simulink model "I_for_8_coils_diagonal_motion"  (R2021b)
settings: Solver=FixedStepAuto  StartTime=4400e-6  StopTime=14760e-6  FixedStep=50e-6  RelTol=1e-3
libraries: simulink x12
(part 2 of 6)

== matlab function I_for_8_coils_diagonal_motion/Left_Coil/Right_Coil/Outer5 Coils/Coil-8 ==
  data: dxp_dz output; x_new input; y_new input; z_new input; dxn_dz output; dyp_dz output; dyn_dz output
function  [dxp_dz, dxn_dz, dyp_dz, dyn_dz] = current(x_new, y_new, z_new)

g = 415e-6;     %Coil spacing
m0 = 4*pi*1e-7;
radius = 3e-3;%m
height = 1e-3;%m
Magentization = 1.45; %T
vol_cy = pi*radius^2*height; % If Object is Cylinder, vol in m^3
% vol_sp = (4/3)*(pi * radius^3); % If Object is Sphere, vol in m^3

k = 0.4e-3; %additional length added to wires, to get concentric coil
%--------%--------%--------%--------%--------%--------%--------%----------
% Line along y - axis
%-%--------%--------%--------%--------%--------%--------%--------%--------
yp1_1 = -0.6e-3 - 7*k;
yp2_1 = 0.6e-3 + 7*k;
yn1_1 = -0.8e-3 - 7*k;
yn2_1 = 0.8e-3 + 7*k;
a_xp_1 = 8*g;  
a_xn_1 = -8*g;

k_yp_1 = 1/(4*pi*((a_xp_1-x_new)^2+z_new^2));
k_1yp_1 = (yp2_1-y_new)/((yp2_1-y_new)^2+(a_xp_1-x_new)^2+z_new^2)^0.5;
k_2yp_1 = (yp1_1-y_new)/((yp1_1-y_new)^2+(a_xp_1-x_new)^2+z_new^2)^0.5;

k_1yp_3 = (yp2_1-y_new)/((yp2_1-y_new)^2+(a_xp_1-x_new)^2+z_new^2)^1.5;
k_2yp_3 = (yp1_1-y_new)/((yp1_1-y_new)^2+(a_xp_1-x_new)^2+z_new^2)^1.5;

k_yn_1 = 1/(4*pi*((a_xn_1-x_new)^2+z_new^2));
k_1yn_1 = (yn2_1-y_new)/((yn2_1-y_new)^2+(a_xn_1-x_new)^2+z_new^2)^0.5;
k_2yn_1 = (yn1_1-y_new)/((yn1_1-y_new)^2+(a_xn_1-x_new)^2+z_new^2)^0.5;

k_1yn_3 = (yn2_1-y_new)/((yn2_1-y_new)^2+(a_xn_1-x_new)^2+z_new^2)^1.5;
k_2yn_3 = (yn1_1-y_new)/((yn1_1-y_new)^2+(a_xn_1-x_new)^2+z_new^2)^1.5;


hyp_z_1 = (k_yp_1) *m0;
hyp_z1_1 = (k_1yp_1 - k_2yp_1)*(-1);
hyp_z2_1 = (k_yp_1*(k_1yp_1 - k_2yp_1)*(z_new^2))*4*pi*2;
hyp_z3_1 = (k_1yp_3 - k_2yp_3)*(z_new^2);
dxp_dz = hyp_z_1*(hyp_z1_1 + hyp_z2_1 + hyp_z3_1);


hyn_z_1 = (k_yn_1)* m0*(-1);
hyn_z1_1 = (k_1yn_1 - k_2yn_1)*(-1);
hyn_z2_1 = (k_yn_1*(k_1yn_1 - k_2yn_1)*(z_new^2))*4*pi*2;
hyn_z3_1 = (k_1yn_3 - k_2yn_3)*(z_new^2);
dxn_dz = hyn_z_1*(hyn_z1_1 + hyn_z2_1 + hyn_z3_1);

%--------%--------%--------%--------%--------%--------%--------%----------
% Line along x - axis
%-%--------%--------%--------%--------%a--------%--------%--------%--------
xp1_1 = -0.8e-3 - 7*k;
xp2_1 = 0.8e-3 + 7*k;
xn1_1 = -1e-3 - 7*k;
xn2_1 = 1e-3 + 7*k;
a_yp_1 = 3.475;          %Distance of coil from (0,0)
a_yn_1 = -3.475;

k_xp_1 = 1/(4*pi*((a_yp_1-y_new)^2+z_new^2));
k_1xp_1 = (xp2_1-x_new)/((xp2_1-x_new)^2+(a_yp_1-y_new)^2+z_new^2)^0.5;
k_2xp_1 = (xp1_1-x_new)/((xp1_1-x_new)^2+(a_yp_1-y_new)^2+z_new^2)^0.5;

k_xn_1 = 1/(4*pi*((a_yn_1-y_new)^2+z_new^2));
k_1xn_1 = (xn2_1-x_new)/((xn2_1-x_new)^2+(a_yn_1-y_new)^2+z_new^2)^0.5;
k_2xn_1 = (xn1_1-x_new)/((xn1_1-x_new)^2+(a_yn_1-y_new)^2+z_new^2)^0.5;

k_1xp_3 = (xp2_1-x_new)/((xp2_1-x_new)^2+(a_yp_1-y_new)^2+z_new^2)^1.5;
k_2xp_3 = (xp1_1-x_new)/((xp1_1-x_new)^2+(a_yp_1-y_new)^2+z_new^2)^1.5;

k_1xn_3 = (xn2_1-x_new)/((xn2_1-x_new)^2+(a_yn_1-y_new)^2+z_new^2)^1.5;
k_2xn_3 = (xn1_1-x_new)/((xn1_1-x_new)^2+(a_yn_1-y_new)^2+z_new^2)^1.5;


hxp_z_1 = (k_xp_1)*m0;
hxp_z1_1 = (k_1xp_1 - k_2xp_1)*(-1);
hxp_z2_1 = (k_xp_1*(k_1xp_1 - k_2xp_1)*(z_new^2))*4*pi*2;
hxp_z3_1 = (k_1xp_3 - k_2xp_3)*(z_new^2);
dyp_dz = hxp_z_1*(hxp_z1_1 + hxp_z2_1 + hxp_z3_1);


hxn_z_1 = (k_xn_1)*m0*(-1);
hxn_z1_1 = (k_1xn_1 - k_2xn_1)*(-1);
hxn_z2_1 = (k_xn_1*(k_1xn_1 - k_2xn_1)*(z_new^2))*4*pi*2;
hxn_z3_1 = (k_1xn_3 - k_2xn_3)*(z_new^2);
dyn_dz = hxn_z_1*(hxn_z1_1 + hxn_z2_1 + hxn_z3_1);

end

== matlab function I_for_8_coils_diagonal_motion/Left_Bottom_Coil/Required Current in Coil1 ==
  data: F_xz_1 input; F_yz_1 input; I output; dxp_dz input; dxn_dz input; dyp_dz input; dyn_dz input; x_new input; y_new input
function  I = current(F_xz_1, F_yz_1,dxp_dz, dxn_dz, dyp_dz, dyn_dz, x_new, y_new)
radius = 3e-3;%m
height = 1e-3;%m
Magentization = 1.45; %T
m0 = 4*pi*10e-7;
vol_cy = pi*radius^2*height; % If Object is Cylinder, vol in m^3
if F_yz_1 == 0 && x_new ~= 0
        I = (F_xz_1/ (dxp_dz + dxn_dz))* m0/ (vol_cy * Magentization);
    elseif F_xz_1 == 0 && y_new ~= 0
        I = (F_yz_1 / (dyp_dz + dyn_dz))* m0/ (vol_cy * Magentization);
    elseif F_xz_1== 0 && F_yz_1 == 0 
        I = 0;
    else
        I = (F_xz_1/ (dxp_dz + dxn_dz)+  F_yz_1 / (dyp_dz + dyn_dz))* m0/ (vol_cy * Magentization);
end
end

== matlab function I_for_8_coils_diagonal_motion/Left_Coil/Right_Coil/Outer5 Coils/Coil-10 ==
  data: dxp_dz output; x_new input; y_new input; z_new input; dxn_dz output; dyp_dz output; dyn_dz output
function  [dxp_dz, dxn_dz, dyp_dz, dyn_dz] = current(x_new, y_new, z_new)

g = 412e-6;     %Coil spacing
m0 = 4*pi*1e-7;
radius = 3e-3;%m
height = 1e-3;%m
Magentization = 1.45; %T
vol_cy = pi*radius^2*height; % If Object is Cylinder, vol in m^3
% vol_sp = (4/3)*(pi * radius^3); % If Object is Sphere, vol in m^3

k = 0.4e-3; %additional length added to wires, to get concentric coil
%--------%--------%--------%--------%--------%--------%--------%----------
% Line along y - axis
%-%--------%--------%--------%--------%--------%--------%--------%--------
yp1_1 = -0.6e-3 - 9*k;
yp2_1 = 0.6e-3 + 9*k;
yn1_1 = -0.8e-3 - 9*k;
yn2_1 = 0.8e-3 + 9*k;
a_xp_1 = 10*g;  
a_xn_1 = -10*g;

k_yp_1 = 1/(4*pi*((a_xp_1-x_new)^2+z_new^2));
k_1yp_1 = (yp2_1-y_new)/((yp2_1-y_new)^2+(a_xp_1-x_new)^2+z_new^2)^0.5;
k_2yp_1 = (yp1_1-y_new)/((yp1_1-y_new)^2+(a_xp_1-x_new)^2+z_new^2)^0.5;

k_1yp_3 = (yp2_1-y_new)/((yp2_1-y_new)^2+(a_xp_1-x_new)^2+z_new^2)^1.5;
k_2yp_3 = (yp1_1-y_new)/((yp1_1-y_new)^2+(a_xp_1-x_new)^2+z_new^2)^1.5;

k_yn_1 = 1/(4*pi*((a_xn_1-x_new)^2+z_new^2));
k_1yn_1 = (yn2_1-y_new)/((yn2_1-y_new)^2+(a_xn_1-x_new)^2+z_new^2)^0.5;
k_2yn_1 = (yn1_1-y_new)/((yn1_1-y_new)^2+(a_xn_1-x_new)^2+z_new^2)^0.5;

k_1yn_3 = (yn2_1-y_new)/((yn2_1-y_new)^2+(a_xn_1-x_new)^2+z_new^2)^1.5;
k_2yn_3 = (yn1_1-y_new)/((yn1_1-y_new)^2+(a_xn_1-x_new)^2+z_new^2)^1.5;


hyp_z_1 = (k_yp_1) *m0;
hyp_z1_1 = (k_1yp_1 - k_2yp_1)*(-1);
hyp_z2_1 = (k_yp_1*(k_1yp_1 - k_2yp_1)*(z_new^2))*4*pi*2;
hyp_z3_1 = (k_1yp_3 - k_2yp_3)*(z_new^2);
dxp_dz = hyp_z_1*(hyp_z1_1 + hyp_z2_1 + hyp_z3_1);


hyn_z_1 = (k_yn_1)* m0*(-1);
hyn_z1_1 = (k_1yn_1 - k_2yn_1)*(-1);
hyn_z2_1 = (k_yn_1*(k_1yn_1 - k_2yn_1)*(z_new^2))*4*pi*2;
hyn_z3_1 = (k_1yn_3 - k_2yn_3)*(z_new^2);
dxn_dz = hyn_z_1*(hyn_z1_1 + hyn_z2_1 + hyn_z3_1);

%--------%--------%--------%--------%--------%--------%--------%----------
% Line along x - axis
%-%--------%--------%--------%--------%a--------%--------%--------%--------
xp1_1 = -0.8e-3 - 9*k;
xp2_1 = 0.8e-3 + 9*k;
xn1_1 = -1e-3 - 9*k;
xn2_1 = 1e-3 + 9*k;
a_yp_1 = 4.275;          %Distance of coil from (0,0)
a_yn_1 = -4.275;

k_xp_1 = 1/(4*pi*((a_yp_1-y_new)^2+z_new^2));
k_1xp_1 = (xp2_1-x_new)/((xp2_1-x_new)^2+(a_yp_1-y_new)^2+z_new^2)^0.5;
k_2xp_1 = (xp1_1-x_new)/((xp1_1-x_new)^2+(a_yp_1-y_new)^2+z_new^2)^0.5;

k_xn_1 = 1/(4*pi*((a_yn_1-y_new)^2+z_new^2));
k_1xn_1 = (xn2_1-x_new)/((xn2_1-x_new)^2+(a_yn_1-y_new)^2+z_new^2)^0.5;
k_2xn_1 = (xn1_1-x_new)/((xn1_1-x_new)^2+(a_yn_1-y_new)^2+z_new^2)^0.5;

k_1xp_3 = (xp2_1-x_new)/((xp2_1-x_new)^2+(a_yp_1-y_new)^2+z_new^2)^1.5;
k_2xp_3 = (xp1_1-x_new)/((xp1_1-x_new)^2+(a_yp_1-y_new)^2+z_new^2)^1.5;

k_1xn_3 = (xn2_1-x_new)/((xn2_1-x_new)^2+(a_yn_1-y_new)^2+z_new^2)^1.5;
k_2xn_3 = (xn1_1-x_new)/((xn1_1-x_new)^2+(a_yn_1-y_new)^2+z_new^2)^1.5;


hxp_z_1 = (k_xp_1)*m0;
hxp_z1_1 = (k_1xp_1 - k_2xp_1)*(-1);
hxp_z2_1 = (k_xp_1*(k_1xp_1 - k_2xp_1)*(z_new^2))*4*pi*2;
hxp_z3_1 = (k_1xp_3 - k_2xp_3)*(z_new^2);
dyp_dz = hxp_z_1*(hxp_z1_1 + hxp_z2_1 + hxp_z3_1);


hxn_z_1 = (k_xn_1)*m0*(-1);
hxn_z1_1 = (k_1xn_1 - k_2xn_1)*(-1);
hxn_z2_1 = (k_xn_1*(k_1xn_1 - k_2xn_1)*(z_new^2))*4*pi*2;
hxn_z3_1 = (k_1xn_3 - k_2xn_3)*(z_new^2);
dyn_dz = hxn_z_1*(hxn_z1_1 + hxn_z2_1 + hxn_z3_1);

end

== matlab function I_for_8_coils_diagonal_motion/Left_Bottom_Coil/Left_Coil/Inner 5 Coils/Coil-1 ==
  data: dxp_dz output; x_new input; y_new input; z_new input; dxn_dz output; dyp_dz output; dyn_dz output
function  [dxp_dz, dxn_dz, dyp_dz, dyn_dz] = current(x_new, y_new, z_new)

g = 520e-6;     %Coil spacing
m0 = 4*pi*1e-7;
radius = 3e-3;%m
height = 1e-3;%m
Magentization = 1.45; %T
vol_cy = pi*radius^2*height; % If Object is Cylinder, vol in m^3
% vol_sp = (4/3)*(pi * radius^3); % If Object is Sphere, vol in m^3

k = 0.4e-3; %additional length added to wires, to get concentric coil
%--------%--------%--------%--------%--------%--------%--------%----------
% Line along y - axis
%-%--------%--------%--------%--------%--------%--------%--------%--------
yp1_1 = -0.6e-3 ;
yp2_1 = 0.6e-3 ;
yn1_1 = -0.8e-3 ;
yn2_1 = 0.8e-3;
a_xp_1 = g;  
a_xn_1 = -g;

k_yp_1 = 1/(4*pi*((a_xp_1-x_new)^2+z_new^2));
k_1yp_1 = (yp2_1-y_new)/((yp2_1-y_new)^2+(a_xp_1-x_new)^2+z_new^2)^0.5;
k_2yp_1 = (yp1_1-y_new)/((yp1_1-y_new)^2+(a_xp_1-x_new)^2+z_new^2)^0.5;

k_1yp_3 = (yp2_1-y_new)/((yp2_1-y_new)^2+(a_xp_1-x_new)^2+z_new^2)^1.5;
k_2yp_3 = (yp1_1-y_new)/((yp1_1-y_new)^2+(a_xp_1-x_new)^2+z_new^2)^1.5;

k_yn_1 = 1/(4*pi*((a_xn_1-x_new)^2+z_new^2));
k_1yn_1 = (yn2_1-y_new)/((yn2_1-y_new)^2+(a_xn_1-x_new)^2+z_new^2)^0.5;
k_2yn_1 = (yn1_1-y_new)/((yn1_1-y_new)^2+(a_xn_1-x_new)^2+z_new^2)^0.5;

k_1yn_3 = (yn2_1-y_new)/((yn2_1-y_new)^2+(a_xn_1-x_new)^2+z_new^2)^1.5;
k_2yn_3 = (yn1_1-y_new)/((yn1_1-y_new)^2+(a_xn_1-x_new)^2+z_new^2)^1.5;


hyp_z_1 = (k_yp_1) *m0;
hyp_z1_1 = (k_1yp_1 - k_2yp_1)*(-1);
hyp_z2_1 = (k_yp_1*(k_1yp_1 - k_2yp_1)*(z_new^2))*4*pi*2;
hyp_z3_1 = (k_1yp_3 - k_2yp_3)*(z_new^2);
dxp_dz = hyp_z_1*(hyp_z1_1 + hyp_z2_1 + hyp_z3_1);


hyn_z_1 = (k_yn_1)* m0*(-1);
hyn_z1_1 = (k_1yn_1 - k_2yn_1)*(-1);
hyn_z2_1 = (k_yn_1*(k_1yn_1 - k_2yn_1)*(z_new^2))*4*pi*2;
hyn_z3_1 = (k_1yn_3 - k_2yn_3)*(z_new^2);
dxn_dz = hyn_z_1*(hyn_z1_1 + hyn_z2_1 + hyn_z3_1);

%--------%--------%--------%--------%--------%--------%--------%----------
% Line along x - axis
%-%--------%--------%--------%--------%a--------%--------%--------%--------
xp1_1 = -0.8e-3 ;
xp2_1 = 0.8e-3 ;
xn1_1 = -1e-3 ;
xn2_1 = 1e-3 ;
a_yp_1 = 0.675;          %Distance of coil from (0,0)
a_yn_1 = -0.675;

k_xp_1 = 1/(4*pi*((a_yp_1-y_new)^2+z_new^2));
k_1xp_1 = (xp2_1-x_new)/((xp2_1-x_new)^2+(a_yp_1-y_new)^2+z_new^2)^0.5;
k_2xp_1 = (xp1_1-x_new)/((xp1_1-x_new)^2+(a_yp_1-y_new)^2+z_new^2)^0.5;

k_xn_1 = 1/(4*pi*((a_yn_1-y_new)^2+z_new^2));
k_1xn_1 = (xn2_1-x_new)/((xn2_1-x_new)^2+(a_yn_1-y_new)^2+z_new^2)^0.5;
k_2xn_1 = (xn1_1-x_new)/((xn1_1-x_new)^2+(a_yn_1-y_new)^2+z_new^2)^0.5;

k_1xp_3 = (xp2_1-x_new)/((xp2_1-x_new)^2+(a_yp_1-y_new)^2+z_new^2)^1.5;
k_2xp_3 = (xp1_1-x_new)/((xp1_1-x_new)^2+(a_yp_1-y_new)^2+z_new^2)^1.5;

k_1xn_3 = (xn2_1-x_new)/((xn2_1-x_new)^2+(a_yn_1-y_new)^2+z_new^2)^1.5;
k_2xn_3 = (xn1_1-x_new)/((xn1_1-x_new)^2+(a_yn_1-y_new)^2+z_new^2)^1.5;


hxp_z_1 = (k_xp_1)*m0;
hxp_z1_1 = (k_1xp_1 - k_2xp_1)*(-1);
hxp_z2_1 = (k_xp_1*(k_1xp_1 - k_2xp_1)*(z_new^2))*4*pi*2;
hxp_z3_1 = (k_1xp_3 - k_2xp_3)*(z_new^2);
dyp_dz = hxp_z_1*(hxp_z1_1 + hxp_z2_1 + hxp_z3_1);


hxn_z_1 = (k_xn_1)*m0*(-1);
hxn_z1_1 = (k_1xn_1 - k_2xn_1)*(-1);
hxn_z2_1 = (k_xn_1*(k_1xn_1 - k_2xn_1)*(z_new^2))*4*pi*2;
hxn_z3_1 = (k_1xn_3 - k_2xn_3)*(z_new^2);
dyn_dz = hxn_z_1*(hxn_z1_1 + hxn_z2_1 + hxn_z3_1);

end

== matlab function I_for_8_coils_diagonal_motion/Left_Bottom_Coil/Left_Coil/Inner 5 Coils/Coil-2 ==
  data: dxp_dz output; x_new input; y_new input; z_new input; dxn_dz output; dyp_dz output; dyn_dz output
function  [dxp_dz, dxn_dz, dyp_dz, dyn_dz] = current(x_new, y_new, z_new)

g = 460e-6;     %Coil spacing
m0 = 4*pi*1e-7;
radius = 3e-3;%m
height = 1e-3;%m
Magentization = 1.45; %T
vol_cy = pi*radius^2*height; % If Object is Cylinder, vol in m^3
% vol_sp = (4/3)*(pi * radius^3); % If Object is Sphere, vol in m^3

k = 0.4e-3; %additional length added to wires, to get concentric coil
%--------%--------%--------%--------%--------%--------%--------%----------
% Line along y - axis
%-%--------%--------%--------%--------%--------%--------%--------%--------
yp1_1 = -0.6e-3 - k;
yp2_1 = 0.6e-3 + k;
yn1_1 = -0.8e-3 - k;
yn2_1 = 0.8e-3 + k;
a_xp_1 = 2*g;  
a_xn_1 = -2*g;

k_yp_1 = 1/(4*pi*((a_xp_1-x_new)^2+z_new^2));
k_1yp_1 = (yp2_1-y_new)/((yp2_1-y_new)^2+(a_xp_1-x_new)^2+z_new^2)^0.5;
k_2yp_1 = (yp1_1-y_new)/((yp1_1-y_new)^2+(a_xp_1-x_new)^2+z_new^2)^0.5;

k_1yp_3 = (yp2_1-y_new)/((yp2_1-y_new)^2+(a_xp_1-x_new)^2+z_new^2)^1.5;
k_2yp_3 = (yp1_1-y_new)/((yp1_1-y_new)^2+(a_xp_1-x_new)^2+z_new^2)^1.5;

k_yn_1 = 1/(4*pi*((a_xn_1-x_new)^2+z_new^2));
k_1yn_1 = (yn2_1-y_new)/((yn2_1-y_new)^2+(a_xn_1-x_new)^2+z_new^2)^0.5;
k_2yn_1 = (yn1_1-y_new)/((yn1_1-y_new)^2+(a_xn_1-x_new)^2+z_new^2)^0.5;

k_1yn_3 = (yn2_1-y_new)/((yn2_1-y_new)^2+(a_xn_1-x_new)^2+z_new^2)^1.5;
k_2yn_3 = (yn1_1-y_new)/((yn1_1-y_new)^2+(a_xn_1-x_new)^2+z_new^2)^1.5;


hyp_z_1 = (k_yp_1) *m0;
hyp_z1_1 = (k_1yp_1 - k_2yp_1)*(-1);
hyp_z2_1 = (k_yp_1*(k_1yp_1 - k_2yp_1)*(z_new^2))*4*pi*2;
hyp_z3_1 = (k_1yp_3 - k_2yp_3)*(z_new^2);
dxp_dz = hyp_z_1*(hyp_z1_1 + hyp_z2_1 + hyp_z3_1);


hyn_z_1 = (k_yn_1)* m0*(-1);
hyn_z1_1 = (k_1yn_1 - k_2yn_1)*(-1);
hyn_z2_1 = (k_yn_1*(k_1yn_1 - k_2yn_1)*(z_new^2))*4*pi*2;
hyn_z3_1 = (k_1yn_3 - k_2yn_3)*(z_new^2);
dxn_dz = hyn_z_1*(hyn_z1_1 + hyn_z2_1 + hyn_z3_1);

%--------%--------%--------%--------%--------%--------%--------%----------
% Line along x - axis
%-%--------%--------%--------%--------%a--------%--------%--------%--------
xp1_1 = -0.8e-3 - k;
xp2_1 = 0.8e-3 + k;
xn1_1 = -1e-3 - k;
xn2_1 = 1e-3 + k;
a_yp_1 = 1.075;          %Distance of coil from (0,0)
a_yn_1 = -1.075;

k_xp_1 = 1/(4*pi*((a_yp_1-y_new)^2+z_new^2));
k_1xp_1 = (xp2_1-x_new)/((xp2_1-x_new)^2+(a_yp_1-y_new)^2+z_new^2)^0.5;
k_2xp_1 = (xp1_1-x_new)/((xp1_1-x_new)^2+(a_yp_1-y_new)^2+z_new^2)^0.5;

k_xn_1 = 1/(4*pi*((a_yn_1-y_new)^2+z_new^2));
k_1xn_1 = (xn2_1-x_new)/((xn2_1-x_new)^2+(a_yn_1-y_new)^2+z_new^2)^0.5;
k_2xn_1 = (xn1_1-x_new)/((xn1_1-x_new)^2+(a_yn_1-y_new)^2+z_new^2)^0.5;

k_1xp_3 = (xp2_1-x_new)/((xp2_1-x_new)^2+(a_yp_1-y_new)^2+z_new^2)^1.5;
k_2xp_3 = (xp1_1-x_new)/((xp1_1-x_new)^2+(a_yp_1-y_new)^2+z_new^2)^1.5;

k_1xn_3 = (xn2_1-x_new)/((xn2_1-x_new)^2+(a_yn_1-y_new)^2+z_new^2)^1.5;
k_2xn_3 = (xn1_1-x_new)/((xn1_1-x_new)^2+(a_yn_1-y_new)^2+z_new^2)^1.5;


hxp_z_1 = (k_xp_1)*m0;
hxp_z1_1 = (k_1xp_1 - k_2xp_1)*(-1);
hxp_z2_1 = (k_xp_1*(k_1xp_1 - k_2xp_1)*(z_new^2))*4*pi*2;
hxp_z3_1 = (k_1xp_3 - k_2xp_3)*(z_new^2);
dyp_dz = hxp_z_1*(hxp_z1_1 + hxp_z2_1 + hxp_z3_1);


hxn_z_1 = (k_xn_1)*m0*(-1);
hxn_z1_1 = (k_1xn_1 - k_2xn_1)*(-1);
hxn_z2_1 = (k_xn_1*(k_1xn_1 - k_2xn_1)*(z_new^2))*4*pi*2;
hxn_z3_1 = (k_1xn_3 - k_2xn_3)*(z_new^2);
dyn_dz = hxn_z_1*(hxn_z1_1 + hxn_z2_1 + hxn_z3_1);

end

== matlab function I_for_8_coils_diagonal_motion/Left_Bottom_Coil/Left_Coil/Inner 5 Coils/Coil-3 ==
  data: dxp_dz output; x_new input; y_new input; z_new input; dxn_dz output; dyp_dz output; dyn_dz output
function  [dxp_dz, dxn_dz, dyp_dz, dyn_dz] = current(x_new, y_new, z_new)

g = 440e-6;     %Coil spacing
m0 = 4*pi*1e-7;
radius = 3e-3;%m
height = 1e-3;%m
Magentization = 1.45; %T
vol_cy = pi*radius^2*height; % If Object is Cylinder, vol in m^3
% vol_sp = (4/3)*(pi * radius^3); % If Object is Sphere, vol in m^3

k = 0.4e-3; %additional length added to wires, to get concentric coil
%--------%--------%--------%--------%--------%--------%--------%----------
% Line along y - axis
%-%--------%--------%--------%--------%--------%--------%--------%--------
yp1_1 = -0.6e-3 - 2*k;
yp2_1 = 0.6e-3 + 2*k;
yn1_1 = -0.8e-3 - 2*k;
yn2_1 = 0.8e-3 + 2*k;
a_xp_1 = 3*g;  
a_xn_1 = -3*g;

k_yp_1 = 1/(4*pi*((a_xp_1-x_new)^2+z_new^2));
k_1yp_1 = (yp2_1-y_new)/((yp2_1-y_new)^2+(a_xp_1-x_new)^2+z_new^2)^0.5;
k_2yp_1 = (yp1_1-y_new)/((yp1_1-y_new)^2+(a_xp_1-x_new)^2+z_new^2)^0.5;

k_1yp_3 = (yp2_1-y_new)/((yp2_1-y_new)^2+(a_xp_1-x_new)^2+z_new^2)^1.5;
k_2yp_3 = (yp1_1-y_new)/((yp1_1-y_new)^2+(a_xp_1-x_new)^2+z_new^2)^1.5;

k_yn_1 = 1/(4*pi*((a_xn_1-x_new)^2+z_new^2));
k_1yn_1 = (yn2_1-y_new)/((yn2_1-y_new)^2+(a_xn_1-x_new)^2+z_new^2)^0.5;
k_2yn_1 = (yn1_1-y_new)/((yn1_1-y_new)^2+(a_xn_1-x_new)^2+z_new^2)^0.5;

k_1yn_3 = (yn2_1-y_new)/((yn2_1-y_new)^2+(a_xn_1-x_new)^2+z_new^2)^1.5;
k_2yn_3 = (yn1_1-y_new)/((yn1_1-y_new)^2+(a_xn_1-x_new)^2+z_new^2)^1.5;


hyp_z_1 = (k_yp_1) *m0;
hyp_z1_1 = (k_1yp_1 - k_2yp_1)*(-1);
hyp_z2_1 = (k_yp_1*(k_1yp_1 - k_2yp_1)*(z_new^2))*4*pi*2;
hyp_z3_1 = (k_1yp_3 - k_2yp_3)*(z_new^2);
dxp_dz = hyp_z_1*(hyp_z1_1 + hyp_z2_1 + hyp_z3_1);


hyn_z_1 = (k_yn_1)* m0*(-1);
hyn_z1_1 = (k_1yn_1 - k_2yn_1)*(-1);
hyn_z2_1 = (k_yn_1*(k_1yn_1 - k_2yn_1)*(z_new^2))*4*pi*2;
hyn_z3_1 = (k_1yn_3 - k_2yn_3)*(z_new^2);
dxn_dz = hyn_z_1*(hyn_z1_1 + hyn_z2_1 + hyn_z3_1);

%--------%--------%--------%--------%--------%--------%--------%----------
% Line along x - axis
%-%--------%--------%--------%--------%a--------%--------%--------%--------
xp1_1 = -0.8e-3 - 2*k;
xp2_1 = 0.8e-3 + 2*k;
xn1_1 = -1e-3 - 2*k;
xn2_1 = 1e-3 + 2*k;
a_yp_1 = 1.475;          %Distance of coil from (0,0)
a_yn_1 = -1.475;

k_xp_1 = 1/(4*pi*((a_yp_1-y_new)^2+z_new^2));
k_1xp_1 = (xp2_1-x_new)/((xp2_1-x_new)^2+(a_yp_1-y_new)^2+z_new^2)^0.5;
k_2xp_1 = (xp1_1-x_new)/((xp1_1-x_new)^2+(a_yp_1-y_new)^2+z_new^2)^0.5;

k_xn_1 = 1/(4*pi*((a_yn_1-y_new)^2+z_new^2));
k_1xn_1 = (xn2_1-x_new)/((xn2_1-x_new)^2+(a_yn_1-y_new)^2+z_new^2)^0.5;
k_2xn_1 = (xn1_1-x_new)/((xn1_1-x_new)^2+(a_yn_1-y_new)^2+z_new^2)^0.5;

k_1xp_3 = (xp2_1-x_new)/((xp2_1-x_new)^2+(a_yp_1-y_new)^2+z_new^2)^1.5;
k_2xp_3 = (xp1_1-x_new)/((xp1_1-x_new)^2+(a_yp_1-y_new)^2+z_new^2)^1.5;

k_1xn_3 = (xn2_1-x_new)/((xn2_1-x_new)^2+(a_yn_1-y_new)^2+z_new^2)^1.5;
k_2xn_3 = (xn1_1-x_new)/((xn1_1-x_new)^2+(a_yn_1-y_new)^2+z_new^2)^1.5;


hxp_z_1 = (k_xp_1)*m0;
hxp_z1_1 = (k_1xp_1 - k_2xp_1)*(-1);
hxp_z2_1 = (k_xp_1*(k_1xp_1 - k_2xp_1)*(z_new^2))*4*pi*2;
hxp_z3_1 = (k_1xp_3 - k_2xp_3)*(z_new^2);
dyp_dz = hxp_z_1*(hxp_z1_1 + hxp_z2_1 + hxp_z3_1);


hxn_z_1 = (k_xn_1)*m0*(-1);
hxn_z1_1 = (k_1xn_1 - k_2xn_1)*(-1);
hxn_z2_1 = (k_xn_1*(k_1xn_1 - k_2xn_1)*(z_new^2))*4*pi*2;
hxn_z3_1 = (k_1xn_3 - k_2xn_3)*(z_new^2);
dyn_dz = hxn_z_1*(hxn_z1_1 + hxn_z2_1 + hxn_z3_1);

end

== matlab function I_for_8_coils_diagonal_motion/Left_Bottom_Coil/Left_Coil/Inner 5 Coils/Coil-4 ==
  data: dxp_dz output; x_new input; y_new input; z_new input; dxn_dz output; dyp_dz output; dyn_dz output
function  [dxp_dz, dxn_dz, dyp_dz, dyn_dz] = current(x_new, y_new, z_new)

g = 430e-6;     %Coil spacing
m0 = 4*pi*1e-7;
radius = 3e-3;%m
height = 1e-3;%m
Magentization = 1.45; %T
vol_cy = pi*radius^2*height; % If Object is Cylinder, vol in m^3
% vol_sp = (4/3)*(pi * radius^3); % If Object is Sphere, vol in m^3

k = 0.4e-3; %additional length added to wires, to get concentric coil
%--------%--------%--------%--------%--------%--------%--------%----------
% Line along y - axis
%-%--------%--------%--------%--------%--------%--------%--------%--------
yp1_1 = -0.6e-3 - 3*k;
yp2_1 = 0.6e-3 + 3*k;
yn1_1 = -0.8e-3 - 3*k;
yn2_1 = 0.8e-3 + 3*k;
a_xp_1 = 4*g;  
a_xn_1 = -4*g;

k_yp_1 = 1/(4*pi*((a_xp_1-x_new)^2+z_new^2));
k_1yp_1 = (yp2_1-y_new)/((yp2_1-y_new)^2+(a_xp_1-x_new)^2+z_new^2)^0.5;
k_2yp_1 = (yp1_1-y_new)/((yp1_1-y_new)^2+(a_xp_1-x_new)^2+z_new^2)^0.5;

k_1yp_3 = (yp2_1-y_new)/((yp2_1-y_new)^2+(a_xp_1-x_new)^2+z_new^2)^1.5;
k_2yp_3 = (yp1_1-y_new)/((yp1_1-y_new)^2+(a_xp_1-x_new)^2+z_new^2)^1.5;

k_yn_1 = 1/(4*pi*((a_xn_1-x_new)^2+z_new^2));
k_1yn_1 = (yn2_1-y_new)/((yn2_1-y_new)^2+(a_xn_1-x_new)^2+z_new^2)^0.5;
k_2yn_1 = (yn1_1-y_new)/((yn1_1-y_new)^2+(a_xn_1-x_new)^2+z_new^2)^0.5;

k_1yn_3 = (yn2_1-y_new)/((yn2_1-y_new)^2+(a_xn_1-x_new)^2+z_new^2)^1.5;
k_2yn_3 = (yn1_1-y_new)/((yn1_1-y_new)^2+(a_xn_1-x_new)^2+z_new^2)^1.5;


hyp_z_1 = (k_yp_1) *m0;
hyp_z1_1 = (k_1yp_1 - k_2yp_1)*(-1);
hyp_z2_1 = (k_yp_1*(k_1yp_1 - k_2yp_1)*(z_new^2))*4*pi*2;
hyp_z3_1 = (k_1yp_3 - k_2yp_3)*(z_new^2);
dxp_dz = hyp_z_1*(hyp_z1_1 + hyp_z2_1 + hyp_z3_1);


hyn_z_1 = (k_yn_1)* m0*(-1);
hyn_z1_1 = (k_1yn_1 - k_2yn_1)*(-1);
hyn_z2_1 = (k_yn_1*(k_1yn_1 - k_2yn_1)*(z_new^2))*4*pi*2;
hyn_z3_1 = (k_1yn_3 - k_2yn_3)*(z_new^2);
dxn_dz = hyn_z_1*(hyn_z1_1 + hyn_z2_1 + hyn_z3_1);

%--------%--------%--------%--------%--------%--------%--------%----------
% Line along x - axis
%-%--------%--------%--------%--------%a--------%--------%--------%--------
xp1_1 = -0.8e-3 - 3*k;
xp2_1 = 0.8e-3 + 3*k;
xn1_1 = -1e-3 - 3*k;
xn2_1 = 1e-3 + 3*k;
a_yp_1 = 1.875;          %Distance of coil from (0,0)
a_yn_1 = -1.875;

k_xp_1 = 1/(4*pi*((a_yp_1-y_new)^2+z_new^2));
k_1xp_1 = (xp2_1-x_new)/((xp2_1-x_new)^2+(a_yp_1-y_new)^2+z_new^2)^0.5;
k_2xp_1 = (xp1_1-x_new)/((xp1_1-x_new)^2+(a_yp_1-y_new)^2+z_new^2)^0.5;

k_xn_1 = 1/(4*pi*((a_yn_1-y_new)^2+z_new^2));
k_1xn_1 = (xn2_1-x_new)/((xn2_1-x_new)^2+(a_yn_1-y_new)^2+z_new^2)^0.5;
k_2xn_1 = (xn1_1-x_new)/((xn1_1-x_new)^2+(a_yn_1-y_new)^2+z_new^2)^0.5;

k_1xp_3 = (xp2_1-x_new)/((xp2_1-x_new)^2+(a_yp_1-y_new)^2+z_new^2)^1.5;
k_2xp_3 = (xp1_1-x_new)/((xp1_1-x_new)^2+(a_yp_1-y_new)^2+z_new^2)^1.5;

k_1xn_3 = (xn2_1-x_new)/((xn2_1-x_new)^2+(a_yn_1-y_new)^2+z_new^2)^1.5;
k_2xn_3 = (xn1_1-x_new)/((xn1_1-x_new)^2+(a_yn_1-y_new)^2+z_new^2)^1.5;


hxp_z_1 = (k_xp_1)*m0;
hxp_z1_1 = (k_1xp_1 - k_2xp_1)*(-1);
hxp_z2_1 = (k_xp_1*(k_1xp_1 - k_2xp_1)*(z_new^2))*4*pi*2;
hxp_z3_1 = (k_1xp_3 - k_2xp_3)*(z_new^2);
dyp_dz = hxp_z_1*(hxp_z1_1 + hxp_z2_1 + hxp_z3_1);


hxn_z_1 = (k_xn_1)*m0*(-1);
hxn_z1_1 = (k_1xn_1 - k_2xn_1)*(-1);
hxn_z2_1 = (k_xn_1*(k_1xn_1 - k_2xn_1)*(z_new^2))*4*pi*2;
hxn_z3_1 = (k_1xn_3 - k_2xn_3)*(z_new^2);
dyn_dz = hxn_z_1*(hxn_z1_1 + hxn_z2_1 + hxn_z3_1);

end

== matlab function I_for_8_coils_diagonal_motion/Left_Bottom_Coil/Left_Coil/Inner 5 Coils/Coil-5 ==
  data: dxp_dz output; x_new input; y_new input; z_new input; dxn_dz output; dyp_dz output; dyn_dz output
function  [dxp_dz, dxn_dz, dyp_dz, dyn_dz] = current(x_new, y_new, z_new)

g = 424e-6;     %Coil spacing
m0 = 4*pi*1e-7;
radius = 3e-3;%m
height = 1e-3;%m
Magentization = 1.45; %T
vol_cy = pi*radius^2*height; % If Object is Cylinder, vol in m^3
% vol_sp = (4/3)*(pi * radius^3); % If Object is Sphere, vol in m^3

k = 0.4e-3; %additional length added to wires, to get concentric coil
%--------%--------%--------%--------%--------%--------%--------%----------
% Line along y - axis
%-%--------%--------%--------%--------%--------%--------%--------%--------
yp1_1 = -0.6e-3 - 4*k;
yp2_1 = 0.6e-3 + 4*k;
yn1_1 = -0.8e-3 - 4*k;
yn2_1 = 0.8e-3 + 4*k;
a_xp_1 = 5*g;  
a_xn_1 = -5*g;

k_yp_1 = 1/(4*pi*((a_xp_1-x_new)^2+z_new^2));
k_1yp_1 = (yp2_1-y_new)/((yp2_1-y_new)^2+(a_xp_1-x_new)^2+z_new^2)^0.5;
k_2yp_1 = (yp1_1-y_new)/((yp1_1-y_new)^2+(a_xp_1-x_new)^2+z_new^2)^0.5;

k_1yp_3 = (yp2_1-y_new)/((yp2_1-y_new)^2+(a_xp_1-x_new)^2+z_new^2)^1.5;
k_2yp_3 = (yp1_1-y_new)/((yp1_1-y_new)^2+(a_xp_1-x_new)^2+z_new^2)^1.5;

k_yn_1 = 1/(4*pi*((a_xn_1-x_new)^2+z_new^2));
k_1yn_1 = (yn2_1-y_new)/((yn2_1-y_new)^2+(a_xn_1-x_new)^2+z_new^2)^0.5;
k_2yn_1 = (yn1_1-y_new)/((yn1_1-y_new)^2+(a_xn_1-x_new)^2+z_new^2)^0.5;

k_1yn_3 = (yn2_1-y_new)/((yn2_1-y_new)^2+(a_xn_1-x_new)^2+z_new^2)^1.5;
k_2yn_3 = (yn1_1-y_new)/((yn1_1-y_new)^2+(a_xn_1-x_new)^2+z_new^2)^1.5;


hyp_z_1 = (k_yp_1) *m0;
hyp_z1_1 = (k_1yp_1 - k_2yp_1)*(-1);
hyp_z2_1 = (k_yp_1*(k_1yp_1 - k_2yp_1)*(z_new^2))*4*pi*2;
hyp_z3_1 = (k_1yp_3 - k_2yp_3)*(z_new^2);
dxp_dz = hyp_z_1*(hyp_z1_1 + hyp_z2_1 + hyp_z3_1);


hyn_z_1 = (k_yn_1)* m0*(-1);
hyn_z1_1 = (k_1yn_1 - k_2yn_1)*(-1);
hyn_z2_1 = (k_yn_1*(k_1yn_1 - k_2yn_1)*(z_new^2))*4*pi*2;
hyn_z3_1 = (k_1yn_3 - k_2yn_3)*(z_new^2);
dxn_dz = hyn_z_1*(hyn_z1_1 + hyn_z2_1 + hyn_z3_1);

%--------%--------%--------%--------%--------%--------%--------%----------
% Line along x - axis
%-%--------%--------%--------%--------%a--------%--------%--------%--------
xp1_1 = -0.8e-3 - 4*k;
xp2_1 = 0.8e-3 + 4*k;
xn1_1 = -1e-3 - 4*k;
xn2_1 = 1e-3 + 4*k;
a_yp_1 = 2.275;          %Distance of coil from (0,0)
a_yn_1 = -2.275;

k_xp_1 = 1/(4*pi*((a_yp_1-y_new)^2+z_new^2));
k_1xp_1 = (xp2_1-x_new)/((xp2_1-x_new)^2+(a_yp_1-y_new)^2+z_new^2)^0.5;
k_2xp_1 = (xp1_1-x_new)/((xp1_1-x_new)^2+(a_yp_1-y_new)^2+z_new^2)^0.5;

k_xn_1 = 1/(4*pi*((a_yn_1-y_new)^2+z_new^2));
k_1xn_1 = (xn2_1-x_new)/((xn2_1-x_new)^2+(a_yn_1-y_new)^2+z_new^2)^0.5;
k_2xn_1 = (xn1_1-x_new)/((xn1_1-x_new)^2+(a_yn_1-y_new)^2+z_new^2)^0.5;

k_1xp_3 = (xp2_1-x_new)/((xp2_1-x_new)^2+(a_yp_1-y_new)^2+z_new^2)^1.5;
k_2xp_3 = (xp1_1-x_new)/((xp1_1-x_new)^2+(a_yp_1-y_new)^2+z_new^2)^1.5;

k_1xn_3 = (xn2_1-x_new)/((xn2_1-x_new)^2+(a_yn_1-y_new)^2+z_new^2)^1.5;
k_2xn_3 = (xn1_1-x_new)/((xn1_1-x_new)^2+(a_yn_1-y_new)^2+z_new^2)^1.5;


hxp_z_1 = (k_xp_1)*m0;
hxp_z1_1 = (k_1xp_1 - k_2xp_1)*(-1);
hxp_z2_1 = (k_xp_1*(k_1xp_1 - k_2xp_1)*(z_new^2))*4*pi*2;
hxp_z3_1 = (k_1xp_3 - k_2xp_3)*(z_new^2);
dyp_dz = hxp_z_1*(hxp_z1_1 + hxp_z2_1 + hxp_z3_1);


hxn_z_1 = (k_xn_1)*m0*(-1);
hxn_z1_1 = (k_1xn_1 - k_2xn_1)*(-1);
hxn_z2_1 = (k_xn_1*(k_1xn_1 - k_2xn_1)*(z_new^2))*4*pi*2;
hxn_z3_1 = (k_1xn_3 - k_2xn_3)*(z_new^2);
dyn_dz = hxn_z_1*(hxn_z1_1 + hxn_z2_1 + hxn_z3_1);

end

== matlab function I_for_8_coils_diagonal_motion/Left_Bottom_Coil/Left_Coil/Outer5 Coils/Coil-10 ==
  data: dxp_dz output; x_new input; y_new input; z_new input; dxn_dz output; dyp_dz output; dyn_dz output
function  [dxp_dz, dxn_dz, dyp_dz, dyn_dz] = current(x_new, y_new, z_new)

g = 412e-6;     %Coil spacing
m0 = 4*pi*1e-7;
radius = 3e-3;%m
height = 1e-3;%m
Magentization = 1.45; %T
vol_cy = pi*radius^2*height; % If Object is Cylinder, vol in m^3
% vol_sp = (4/3)*(pi * radius^3); % If Object is Sphere, vol in m^3

k = 0.4e-3; %additional length added to wires, to get concentric coil
%--------%--------%--------%--------%--------%--------%--------%----------
% Line along y - axis
%-%--------%--------%--------%--------%--------%--------%--------%--------
yp1_1 = -0.6e-3 - 9*k;
yp2_1 = 0.6e-3 + 9*k;
yn1_1 = -0.8e-3 - 9*k;
yn2_1 = 0.8e-3 + 9*k;
a_xp_1 = 10*g;  
a_xn_1 = -10*g;

k_yp_1 = 1/(4*pi*((a_xp_1-x_new)^2+z_new^2));
k_1yp_1 = (yp2_1-y_new)/((yp2_1-y_new)^2+(a_xp_1-x_new)^2+z_new^2)^0.5;
k_2yp_1 = (yp1_1-y_new)/((yp1_1-y_new)^2+(a_xp_1-x_new)^2+z_new^2)^0.5;

k_1yp_3 = (yp2_1-y_new)/((yp2_1-y_new)^2+(a_xp_1-x_new)^2+z_new^2)^1.5;
k_2yp_3 = (yp1_1-y_new)/((yp1_1-y_new)^2+(a_xp_1-x_new)^2+z_new^2)^1.5;

k_yn_1 = 1/(4*pi*((a_xn_1-x_new)^2+z_new^2));
k_1yn_1 = (yn2_1-y_new)/((yn2_1-y_new)^2+(a_xn_1-x_new)^2+z_new^2)^0.5;
k_2yn_1 = (yn1_1-y_new)/((yn1_1-y_new)^2+(a_xn_1-x_new)^2+z_new^2)^0.5;

k_1yn_3 = (yn2_1-y_new)/((yn2_1-y_new)^2+(a_xn_1-x_new)^2+z_new^2)^1.5;
k_2yn_3 = (yn1_1-y_new)/((yn1_1-y_new)^2+(a_xn_1-x_new)^2+z_new^2)^1.5;


hyp_z_1 = (k_yp_1) *m0;
hyp_z1_1 = (k_1yp_1 - k_2yp_1)*(-1);
hyp_z2_1 = (k_yp_1*(k_1yp_1 - k_2yp_1)*(z_new^2))*4*pi*2;
hyp_z3_1 = (k_1yp_3 - k_2yp_3)*(z_new^2);
dxp_dz = hyp_z_1*(hyp_z1_1 + hyp_z2_1 + hyp_z3_1);


hyn_z_1 = (k_yn_1)* m0*(-1);
hyn_z1_1 = (k_1yn_1 - k_2yn_1)*(-1);
hyn_z2_1 = (k_yn_1*(k_1yn_1 - k_2yn_1)*(z_new^2))*4*pi*2;
hyn_z3_1 = (k_1yn_3 - k_2yn_3)*(z_new^2);
dxn_dz = hyn_z_1*(hyn_z1_1 + hyn_z2_1 + hyn_z3_1);

%--------%--------%--------%--------%--------%--------%--------%----------
% Line along x - axis
%-%--------%--------%--------%--------%a--------%--------%--------%--------
xp1_1 = -0.8e-3 - 9*k;
xp2_1 = 0.8e-3 + 9*k;
xn1_1 = -1e-3 - 9*k;
xn2_1 = 1e-3 + 9*k;
a_yp_1 = 4.275;          %Distance of coil from (0,0)
a_yn_1 = -4.275;

k_xp_1 = 1/(4*pi*((a_yp_1-y_new)^2+z_new^2));
k_1xp_1 = (xp2_1-x_new)/((xp2_1-x_new)^2+(a_yp_1-y_new)^2+z_new^2)^0.5;
k_2xp_1 = (xp1_1-x_new)/((xp1_1-x_new)^2+(a_yp_1-y_new)^2+z_new^2)^0.5;

k_xn_1 = 1/(4*pi*((a_yn_1-y_new)^2+z_new^2));
k_1xn_1 = (xn2_1-x_new)/((xn2_1-x_new)^2+(a_yn_1-y_new)^2+z_new^2)^0.5;
k_2xn_1 = (xn1_1-x_new)/((xn1_1-x_new)^2+(a_yn_1-y_new)^2+z_new^2)^0.5;

k_1xp_3 = (xp2_1-x_new)/((xp2_1-x_new)^2+(a_yp_1-y_new)^2+z_new^2)^1.5;
k_2xp_3 = (xp1_1-x_new)/((xp1_1-x_new)^2+(a_yp_1-y_new)^2+z_new^2)^1.5;

k_1xn_3 = (xn2_1-x_new)/((xn2_1-x_new)^2+(a_yn_1-y_new)^2+z_new^2)^1.5;
k_2xn_3 = (xn1_1-x_new)/((xn1_1-x_new)^2+(a_yn_1-y_new)^2+z_new^2)^1.5;


hxp_z_1 = (k_xp_1)*m0;
hxp_z1_1 = (k_1xp_1 - k_2xp_1)*(-1);
hxp_z2_1 = (k_xp_1*(k_1xp_1 - k_2xp_1)*(z_new^2))*4*pi*2;
hxp_z3_1 = (k_1xp_3 - k_2xp_3)*(z_new^2);
dyp_dz = hxp_z_1*(hxp_z1_1 + hxp_z2_1 + hxp_z3_1);


hxn_z_1 = (k_xn_1)*m0*(-1);
hxn_z1_1 = (k_1xn_1 - k_2xn_1)*(-1);
hxn_z2_1 = (k_xn_1*(k_1xn_1 - k_2xn_1)*(z_new^2))*4*pi*2;
hxn_z3_1 = (k_1xn_3 - k_2xn_3)*(z_new^2);
dyn_dz = hxn_z_1*(hxn_z1_1 + hxn_z2_1 + hxn_z3_1);

end

== matlab function I_for_8_coils_diagonal_motion/Left_Coil/Right_Coil/Inner 5 Coils/Coil-1 ==
  data: dxp_dz output; x_new input; y_new input; z_new input; dxn_dz output; dyp_dz output; dyn_dz output
function  [dxp_dz, dxn_dz, dyp_dz, dyn_dz] = current(x_new, y_new, z_new)

g = 520e-6;     %Coil spacing
m0 = 4*pi*1e-7;
radius = 3e-3;%m
height = 1e-3;%m
Magentization = 1.45; %T
vol_cy = pi*radius^2*height; % If Object is Cylinder, vol in m^3
% vol_sp = (4/3)*(pi * radius^3); % If Object is Sphere, vol in m^3

k = 0.4e-3; %additional length added to wires, to get concentric coil
%--------%--------%--------%--------%--------%--------%--------%----------
% Line along y - axis
%-%--------%--------%--------%--------%--------%--------%--------%--------
yp1_1 = -0.6e-3 ;
yp2_1 = 0.6e-3 ;
yn1_1 = -0.8e-3 ;
yn2_1 = 0.8e-3;
a_xp_1 = g;  
a_xn_1 = -g;

k_yp_1 = 1/(4*pi*((a_xp_1-x_new)^2+z_new^2));
k_1yp_1 = (yp2_1-y_new)/((yp2_1-y_new)^2+(a_xp_1-x_new)^2+z_new^2)^0.5;
k_2yp_1 = (yp1_1-y_new)/((yp1_1-y_new)^2+(a_xp_1-x_new)^2+z_new^2)^0.5;

k_1yp_3 = (yp2_1-y_new)/((yp2_1-y_new)^2+(a_xp_1-x_new)^2+z_new^2)^1.5;
k_2yp_3 = (yp1_1-y_new)/((yp1_1-y_new)^2+(a_xp_1-x_new)^2+z_new^2)^1.5;

k_yn_1 = 1/(4*pi*((a_xn_1-x_new)^2+z_new^2));
k_1yn_1 = (yn2_1-y_new)/((yn2_1-y_new)^2+(a_xn_1-x_new)^2+z_new^2)^0.5;
k_2yn_1 = (yn1_1-y_new)/((yn1_1-y_new)^2+(a_xn_1-x_new)^2+z_new^2)^0.5;

k_1yn_3 = (yn2_1-y_new)/((yn2_1-y_new)^2+(a_xn_1-x_new)^2+z_new^2)^1.5;
k_2yn_3 = (yn1_1-y_new)/((yn1_1-y_new)^2+(a_xn_1-x_new)^2+z_new^2)^1.5;


hyp_z_1 = (k_yp_1) *m0;
hyp_z1_1 = (k_1yp_1 - k_2yp_1)*(-1);
hyp_z2_1 = (k_yp_1*(k_1yp_1 - k_2yp_1)*(z_new^2))*4*pi*2;
hyp_z3_1 = (k_1yp_3 - k_2yp_3)*(z_new^2);
dxp_dz = hyp_z_1*(hyp_z1_1 + hyp_z2_1 + hyp_z3_1);


hyn_z_1 = (k_yn_1)* m0*(-1);
hyn_z1_1 = (k_1yn_1 - k_2yn_1)*(-1);
hyn_z2_1 = (k_yn_1*(k_1yn_1 - k_2yn_1)*(z_new^2))*4*pi*2;
hyn_z3_1 = (k_1yn_3 - k_2yn_3)*(z_new^2);
dxn_dz = hyn_z_1*(hyn_z1_1 + hyn_z2_1 + hyn_z3_1);

%--------%--------%--------%--------%--------%--------%--------%----------
% Line along x - axis
%-%--------%--------%--------%--------%a--------%--------%--------%--------
xp1_1 = -0.8e-3 ;
xp2_1 = 0.8e-3 ;
xn1_1 = -1e-3 ;
xn2_1 = 1e-3 ;
a_yp_1 = 0.675;          %Distance of coil from (0,0)
a_yn_1 = -0.675;

k_xp_1 = 1/(4*pi*((a_yp_1-y_new)^2+z_new^2));
k_1xp_1 = (xp2_1-x_new)/((xp2_1-x_new)^2+(a_yp_1-y_new)^2+z_new^2)^0.5;
k_2xp_1 = (xp1_1-x_new)/((xp1_1-x_new)^2+(a_yp_1-y_new)^2+z_new^2)^0.5;

k_xn_1 = 1/(4*pi*((a_yn_1-y_new)^2+z_new^2));
k_1xn_1 = (xn2_1-x_new)/((xn2_1-x_new)^2+(a_yn_1-y_new)^2+z_new^2)^0.5;
k_2xn_1 = (xn1_1-x_new)/((xn1_1-x_new)^2+(a_yn_1-y_new)^2+z_new^2)^0.5;

k_1xp_3 = (xp2_1-x_new)/((xp2_1-x_new)^2+(a_yp_1-y_new)^2+z_new^2)^1.5;
k_2xp_3 = (xp1_1-x_new)/((xp1_1-x_new)^2+(a_yp_1-y_new)^2+z_new^2)^1.5;

k_1xn_3 = (xn2_1-x_new)/((xn2_1-x_new)^2+(a_yn_1-y_new)^2+z_new^2)^1.5;
k_2xn_3 = (xn1_1-x_new)/((xn1_1-x_new)^2+(a_yn_1-y_new)^2+z_new^2)^1.5;


hxp_z_1 = (k_xp_1)*m0;
hxp_z1_1 = (k_1xp_1 - k_2xp_1)*(-1);
hxp_z2_1 = (k_xp_1*(k_1xp_1 - k_2xp_1)*(z_new^2))*4*pi*2;
hxp_z3_1 = (k_1xp_3 - k_2xp_3)*(z_new^2);
dyp_dz = hxp_z_1*(hxp_z1_1 + hxp_z2_1 + hxp_z3_1);


hxn_z_1 = (k_xn_1)*m0*(-1);
hxn_z1_1 = (k_1xn_1 - k_2xn_1)*(-1);
hxn_z2_1 = (k_xn_1*(k_1xn_1 - k_2xn_1)*(z_new^2))*4*pi*2;
hxn_z3_1 = (k_1xn_3 - k_2xn_3)*(z_new^2);
dyn_dz = hxn_z_1*(hxn_z1_1 + hxn_z2_1 + hxn_z3_1);

end

== matlab function I_for_8_coils_diagonal_motion/Left_Bottom_Coil/Left_Coil/Outer5 Coils/Coil-6 ==
  data: dxp_dz output; x_new input; y_new input; z_new input; dxn_dz output; dyp_dz output; dyn_dz output
function  [dxp_dz, dxn_dz, dyp_dz, dyn_dz] = current(x_new, y_new, z_new)

g = 420e-6;     %Coil spacing
m0 = 4*pi*1e-7;
radius = 3e-3;%m
height = 1e-3;%m
Magentization = 1.45; %T
vol_cy = pi*radius^2*height; % If Object is Cylinder, vol in m^3
% vol_sp = (4/3)*(pi * radius^3); % If Object is Sphere, vol in m^3

k = 0.4e-3; %additional length added to wires, to get concentric coil
%--------%--------%--------%--------%--------%--------%--------%----------
% Line along y - axis
%-%--------%--------%--------%--------%--------%--------%--------%--------
yp1_1 = -0.6e-3 - 5*k;
yp2_1 = 0.6e-3 + 5*k;
yn1_1 = -0.8e-3 - 5*k;
yn2_1 = 0.8e-3 + 5*k;
a_xp_1 = 6*g;  
a_xn_1 = -6*g;

k_yp_1 = 1/(4*pi*((a_xp_1-x_new)^2+z_new^2));
k_1yp_1 = (yp2_1-y_new)/((yp2_1-y_new)^2+(a_xp_1-x_new)^2+z_new^2)^0.5;
k_2yp_1 = (yp1_1-y_new)/((yp1_1-y_new)^2+(a_xp_1-x_new)^2+z_new^2)^0.5;

k_1yp_3 = (yp2_1-y_new)/((yp2_1-y_new)^2+(a_xp_1-x_new)^2+z_new^2)^1.5;
k_2yp_3 = (yp1_1-y_new)/((yp1_1-y_new)^2+(a_xp_1-x_new)^2+z_new^2)^1.5;

k_yn_1 = 1/(4*pi*((a_xn_1-x_new)^2+z_new^2));
k_1yn_1 = (yn2_1-y_new)/((yn2_1-y_new)^2+(a_xn_1-x_new)^2+z_new^2)^0.5;
k_2yn_1 = (yn1_1-y_new)/((yn1_1-y_new)^2+(a_xn_1-x_new)^2+z_new^2)^0.5;

k_1yn_3 = (yn2_1-y_new)/((yn2_1-y_new)^2+(a_xn_1-x_new)^2+z_new^2)^1.5;
k_2yn_3 = (yn1_1-y_new)/((yn1_1-y_new)^2+(a_xn_1-x_new)^2+z_new^2)^1.5;


hyp_z_1 = (k_yp_1) *m0;
hyp_z1_1 = (k_1yp_1 - k_2yp_1)*(-1);
hyp_z2_1 = (k_yp_1*(k_1yp_1 - k_2yp_1)*(z_new^2))*4*pi*2;
hyp_z3_1 = (k_1yp_3 - k_2yp_3)*(z_new^2);
dxp_dz = hyp_z_1*(hyp_z1_1 + hyp_z2_1 + hyp_z3_1);


hyn_z_1 = (k_yn_1)* m0*(-1);
hyn_z1_1 = (k_1yn_1 - k_2yn_1)*(-1);
hyn_z2_1 = (k_yn_1*(k_1yn_1 - k_2yn_1)*(z_new^2))*4*pi*2;
hyn_z3_1 = (k_1yn_3 - k_2yn_3)*(z_new^2);
dxn_dz = hyn_z_1*(hyn_z1_1 + hyn_z2_1 + hyn_z3_1);

%--------%--------%--------%--------%--------%--------%--------%----------
% Line along x - axis
%-%--------%--------%--------%--------%a--------%--------%--------%--------
xp1_1 = -0.8e-3 - 5*k;
xp2_1 = 0.8e-3 + 5*k;
xn1_1 = -1e-3 - 5*k;
xn2_1 = 1e-3 + 5*k;
a_yp_1 = 2.675;          %Distance of coil from (0,0)
a_yn_1 = -2.675;

k_xp_1 = 1/(4*pi*((a_yp_1-y_new)^2+z_new^2));
k_1xp_1 = (xp2_1-x_new)/((xp2_1-x_new)^2+(a_yp_1-y_new)^2+z_new^2)^0.5;
k_2xp_1 = (xp1_1-x_new)/((xp1_1-x_new)^2+(a_yp_1-y_new)^2+z_new^2)^0.5;

k_xn_1 = 1/(4*pi*((a_yn_1-y_new)^2+z_new^2));
k_1xn_1 = (xn2_1-x_new)/((xn2_1-x_new)^2+(a_yn_1-y_new)^2+z_new^2)^0.5;
k_2xn_1 = (xn1_1-x_new)/((xn1_1-x_new)^2+(a_yn_1-y_new)^2+z_new^2)^0.5;

k_1xp_3 = (xp2_1-x_new)/((xp2_1-x_new)^2+(a_yp_1-y_new)^2+z_new^2)^1.5;
k_2xp_3 = (xp1_1-x_new)/((xp1_1-x_new)^2+(a_yp_1-y_new)^2+z_new^2)^1.5;

k_1xn_3 = (xn2_1-x_new)/((xn2_1-x_new)^2+(a_yn_1-y_new)^2+z_new^2)^1.5;
k_2xn_3 = (xn1_1-x_new)/((xn1_1-x_new)^2+(a_yn_1-y_new)^2+z_new^2)^1.5;


hxp_z_1 = (k_xp_1)*m0;
hxp_z1_1 = (k_1xp_1 - k_2xp_1)*(-1);
hxp_z2_1 = (k_xp_1*(k_1xp_1 - k_2xp_1)*(z_new^2))*4*pi*2;
hxp_z3_1 = (k_1xp_3 - k_2xp_3)*(z_new^2);
dyp_dz = hxp_z_1*(hxp_z1_1 + hxp_z2_1 + hxp_z3_1);


hxn_z_1 = (k_xn_1)*m0*(-1);
hxn_z1_1 = (k_1xn_1 - k_2xn_1)*(-1);
hxn_z2_1 = (k_xn_1*(k_1xn_1 - k_2xn_1)*(z_new^2))*4*pi*2;
hxn_z3_1 = (k_1xn_3 - k_2xn_3)*(z_new^2);
dyn_dz = hxn_z_1*(hxn_z1_1 + hxn_z2_1 + hxn_z3_1);

end

== matlab function I_for_8_coils_diagonal_motion/Left_Bottom_Coil/Left_Coil/Outer5 Coils/Coil-7 ==
  data: dxp_dz output; x_new input; y_new input; z_new input; dxn_dz output; dyp_dz output; dyn_dz output
function  [dxp_dz, dxn_dz, dyp_dz, dyn_dz] = current(x_new, y_new, z_new)

g = 417.14e-6;     %Coil spacing
m0 = 4*pi*1e-7;
radius = 3e-3;%m
height = 1e-3;%m
Magentization = 1.45; %T
vol_cy = pi*radius^2*height; % If Object is Cylinder, vol in m^3
% vol_sp = (4/3)*(pi * radius^3); % If Object is Sphere, vol in m^3

k = 0.4e-3; %additional length added to wires, to get concentric coil
%--------%--------%--------%--------%--------%--------%--------%----------
% Line along y - axis
%-%--------%--------%--------%--------%--------%--------%--------%--------
yp1_1 = -0.6e-3 - 6*k;
yp2_1 = 0.6e-3 + 6*k;
yn1_1 = -0.8e-3 - 6*k;
yn2_1 = 0.8e-3 + 6*k;
a_xp_1 = 7*g;  
a_xn_1 = -7*g;

k_yp_1 = 1/(4*pi*((a_xp_1-x_new)^2+z_new^2));
k_1yp_1 = (yp2_1-y_new)/((yp2_1-y_new)^2+(a_xp_1-x_new)^2+z_new^2)^0.5;
k_2yp_1 = (yp1_1-y_new)/((yp1_1-y_new)^2+(a_xp_1-x_new)^2+z_new^2)^0.5;

k_1yp_3 = (yp2_1-y_new)/((yp2_1-y_new)^2+(a_xp_1-x_new)^2+z_new^2)^1.5;
k_2yp_3 = (yp1_1-y_new)/((yp1_1-y_new)^2+(a_xp_1-x_new)^2+z_new^2)^1.5;

k_yn_1 = 1/(4*pi*((a_xn_1-x_new)^2+z_new^2));
k_1yn_1 = (yn2_1-y_new)/((yn2_1-y_new)^2+(a_xn_1-x_new)^2+z_new^2)^0.5;
k_2yn_1 = (yn1_1-y_new)/((yn1_1-y_new)^2+(a_xn_1-x_new)^2+z_new^2)^0.5;

k_1yn_3 = (yn2_1-y_new)/((yn2_1-y_new)^2+(a_xn_1-x_new)^2+z_new^2)^1.5;
k_2yn_3 = (yn1_1-y_new)/((yn1_1-y_new)^2+(a_xn_1-x_new)^2+z_new^2)^1.5;


hyp_z_1 = (k_yp_1) *m0;
hyp_z1_1 = (k_1yp_1 - k_2yp_1)*(-1);
hyp_z2_1 = (k_yp_1*(k_1yp_1 - k_2yp_1)*(z_new^2))*4*pi*2;
hyp_z3_1 = (k_1yp_3 - k_2yp_3)*(z_new^2);
dxp_dz = hyp_z_1*(hyp_z1_1 + hyp_z2_1 + hyp_z3_1);


hyn_z_1 = (k_yn_1)* m0*(-1);
hyn_z1_1 = (k_1yn_1 - k_2yn_1)*(-1);
hyn_z2_1 = (k_yn_1*(k_1yn_1 - k_2yn_1)*(z_new^2))*4*pi*2;
hyn_z3_1 = (k_1yn_3 - k_2yn_3)*(z_new^2);
dxn_dz = hyn_z_1*(hyn_z1_1 + hyn_z2_1 + hyn_z3_1);

%--------%--------%--------%--------%--------%--------%--------%----------
% Line along x - axis
%-%--------%--------%--------%--------%a--------%--------%--------%--------
xp1_1 = -0.8e-3 - 6*k;
xp2_1 = 0.8e-3 + 6*k;
xn1_1 = -1e-3 - 6*k;
xn2_1 = 1e-3 + 6*k;
a_yp_1 = 3.075;          %Distance of coil from (0,0)
a_yn_1 = -3.075;

k_xp_1 = 1/(4*pi*((a_yp_1-y_new)^2+z_new^2));
k_1xp_1 = (xp2_1-x_new)/((xp2_1-x_new)^2+(a_yp_1-y_new)^2+z_new^2)^0.5;
k_2xp_1 = (xp1_1-x_new)/((xp1_1-x_new)^2+(a_yp_1-y_new)^2+z_new^2)^0.5;

k_xn_1 = 1/(4*pi*((a_yn_1-y_new)^2+z_new^2));
k_1xn_1 = (xn2_1-x_new)/((xn2_1-x_new)^2+(a_yn_1-y_new)^2+z_new^2)^0.5;
k_2xn_1 = (xn1_1-x_new)/((xn1_1-x_new)^2+(a_yn_1-y_new)^2+z_new^2)^0.5;

k_1xp_3 = (xp2_1-x_new)/((xp2_1-x_new)^2+(a_yp_1-y_new)^2+z_new^2)^1.5;
k_2xp_3 = (xp1_1-x_new)/((xp1_1-x_new)^2+(a_yp_1-y_new)^2+z_new^2)^1.5;

k_1xn_3 = (xn2_1-x_new)/((xn2_1-x_new)^2+(a_yn_1-y_new)^2+z_new^2)^1.5;
k_2xn_3 = (xn1_1-x_new)/((xn1_1-x_new)^2+(a_yn_1-y_new)^2+z_new^2)^1.5;


hxp_z_1 = (k_xp_1)*m0;
hxp_z1_1 = (k_1xp_1 - k_2xp_1)*(-1);
hxp_z2_1 = (k_xp_1*(k_1xp_1 - k_2xp_1)*(z_new^2))*4*pi*2;
hxp_z3_1 = (k_1xp_3 - k_2xp_3)*(z_new^2);
dyp_dz = hxp_z_1*(hxp_z1_1 + hxp_z2_1 + hxp_z3_1);


hxn_z_1 = (k_xn_1)*m0*(-1);
hxn_z1_1 = (k_1xn_1 - k_2xn_1)*(-1);
hxn_z2_1 = (k_xn_1*(k_1xn_1 - k_2xn_1)*(z_new^2))*4*pi*2;
hxn_z3_1 = (k_1xn_3 - k_2xn_3)*(z_new^2);
dyn_dz = hxn_z_1*(hxn_z1_1 + hxn_z2_1 + hxn_z3_1);

end

== matlab function I_for_8_coils_diagonal_motion/Left_Bottom_Coil/Left_Coil/Outer5 Coils/Coil-8 ==
  data: dxp_dz output; x_new input; y_new input; z_new input; dxn_dz output; dyp_dz output; dyn_dz output
function  [dxp_dz, dxn_dz, dyp_dz, dyn_dz] = current(x_new, y_new, z_new)

g = 415e-6;     %Coil spacing
m0 = 4*pi*1e-7;
radius = 3e-3;%m
height = 1e-3;%m
Magentization = 1.45; %T
vol_cy = pi*radius^2*height; % If Object is Cylinder, vol in m^3
% vol_sp = (4/3)*(pi * radius^3); % If Object is Sphere, vol in m^3

k = 0.4e-3; %additional length added to wires, to get concentric coil
%--------%--------%--------%--------%--------%--------%--------%----------
% Line along y - axis
%-%--------%--------%--------%--------%--------%--------%--------%--------
yp1_1 = -0.6e-3 - 7*k;
yp2_1 = 0.6e-3 + 7*k;
yn1_1 = -0.8e-3 - 7*k;
yn2_1 = 0.8e-3 + 7*k;
a_xp_1 = 8*g;  
a_xn_1 = -8*g;

k_yp_1 = 1/(4*pi*((a_xp_1-x_new)^2+z_new^2));
k_1yp_1 = (yp2_1-y_new)/((yp2_1-y_new)^2+(a_xp_1-x_new)^2+z_new^2)^0.5;
k_2yp_1 = (yp1_1-y_new)/((yp1_1-y_new)^2+(a_xp_1-x_new)^2+z_new^2)^0.5;

k_1yp_3 = (yp2_1-y_new)/((yp2_1-y_new)^2+(a_xp_1-x_new)^2+z_new^2)^1.5;
k_2yp_3 = (yp1_1-y_new)/((yp1_1-y_new)^2+(a_xp_1-x_new)^2+z_new^2)^1.5;

k_yn_1 = 1/(4*pi*((a_xn_1-x_new)^2+z_new^2));
k_1yn_1 = (yn2_1-y_new)/((yn2_1-y_new)^2+(a_xn_1-x_new)^2+z_new^2)^0.5;
k_2yn_1 = (yn1_1-y_new)/((yn1_1-y_new)^2+(a_xn_1-x_new)^2+z_new^2)^0.5;

k_1yn_3 = (yn2_1-y_new)/((yn2_1-y_new)^2+(a_xn_1-x_new)^2+z_new^2)^1.5;
k_2yn_3 = (yn1_1-y_new)/((yn1_1-y_new)^2+(a_xn_1-x_new)^2+z_new^2)^1.5;


hyp_z_1 = (k_yp_1) *m0;
hyp_z1_1 = (k_1yp_1 - k_2yp_1)*(-1);
hyp_z2_1 = (k_yp_1*(k_1yp_1 - k_2yp_1)*(z_new^2))*4*pi*2;
hyp_z3_1 = (k_1yp_3 - k_2yp_3)*(z_new^2);
dxp_dz = hyp_z_1*(hyp_z1_1 + hyp_z2_1 + hyp_z3_1);


hyn_z_1 = (k_yn_1)* m0*(-1);
hyn_z1_1 = (k_1yn_1 - k_2yn_1)*(-1);
hyn_z2_1 = (k_yn_1*(k_1yn_1 - k_2yn_1)*(z_new^2))*4*pi*2;
hyn_z3_1 = (k_1yn_3 - k_2yn_3)*(z_new^2);
dxn_dz = hyn_z_1*(hyn_z1_1 + hyn_z2_1 + hyn_z3_1);

%--------%--------%--------%--------%--------%--------%--------%----------
% Line along x - axis
%-%--------%--------%--------%--------%a--------%--------%--------%--------
xp1_1 = -0.8e-3 - 7*k;
xp2_1 = 0.8e-3 + 7*k;
xn1_1 = -1e-3 - 7*k;
xn2_1 = 1e-3 + 7*k;
a_yp_1 = 3.475;          %Distance of coil from (0,0)
a_yn_1 = -3.475;

k_xp_1 = 1/(4*pi*((a_yp_1-y_new)^2+z_new^2));
k_1xp_1 = (xp2_1-x_new)/((xp2_1-x_new)^2+(a_yp_1-y_new)^2+z_new^2)^0.5;
k_2xp_1 = (xp1_1-x_new)/((xp1_1-x_new)^2+(a_yp_1-y_new)^2+z_new^2)^0.5;

k_xn_1 = 1/(4*pi*((a_yn_1-y_new)^2+z_new^2));
k_1xn_1 = (xn2_1-x_new)/((xn2_1-x_new)^2+(a_yn_1-y_new)^2+z_new^2)^0.5;
k_2xn_1 = (xn1_1-x_new)/((xn1_1-x_new)^2+(a_yn_1-y_new)^2+z_new^2)^0.5;

k_1xp_3 = (xp2_1-x_new)/((xp2_1-x_new)^2+(a_yp_1-y_new)^2+z_new^2)^1.5;
k_2xp_3 = (xp1_1-x_new)/((xp1_1-x_new)^2+(a_yp_1-y_new)^2+z_new^2)^1.5;

k_1xn_3 = (xn2_1-x_new)/((xn2_1-x_new)^2+(a_yn_1-y_new)^2+z_new^2)^1.5;
k_2xn_3 = (xn1_1-x_new)/((xn1_1-x_new)^2+(a_yn_1-y_new)^2+z_new^2)^1.5;


hxp_z_1 = (k_xp_1)*m0;
hxp_z1_1 = (k_1xp_1 - k_2xp_1)*(-1);
hxp_z2_1 = (k_xp_1*(k_1xp_1 - k_2xp_1)*(z_new^2))*4*pi*2;
hxp_z3_1 = (k_1xp_3 - k_2xp_3)*(z_new^2);
dyp_dz = hxp_z_1*(hxp_z1_1 + hxp_z2_1 + hxp_z3_1);


hxn_z_1 = (k_xn_1)*m0*(-1);
hxn_z1_1 = (k_1xn_1 - k_2xn_1)*(-1);
hxn_z2_1 = (k_xn_1*(k_1xn_1 - k_2xn_1)*(z_new^2))*4*pi*2;
hxn_z3_1 = (k_1xn_3 - k_2xn_3)*(z_new^2);
dyn_dz = hxn_z_1*(hxn_z1_1 + hxn_z2_1 + hxn_z3_1);

end

== matlab function I_for_8_coils_diagonal_motion/Left_Bottom_Coil/Left_Coil/Outer5 Coils/Coil-9 ==
  data: dxp_dz output; x_new input; y_new input; z_new input; dxn_dz output; dyp_dz output; dyn_dz output
function  [dxp_dz, dxn_dz, dyp_dz, dyn_dz] = current(x_new, y_new, z_new)

g = 415e-6;     %Coil spacing
m0 = 4*pi*1e-7;
radius = 3e-3;%m
height = 1e-3;%m
Magentization = 1.45; %T
vol_cy = pi*radius^2*height; % If Object is Cylinder, vol in m^3
% vol_sp = (4/3)*(pi * radius^3); % If Object is Sphere, vol in m^3

k = 0.4e-3; %additional length added to wires, to get concentric coil
%--------%--------%--------%--------%--------%--------%--------%----------
% Line along y - axis
%-%--------%--------%--------%--------%--------%--------%--------%--------
yp1_1 = -0.6e-3 - 8*k;
yp2_1 = 0.6e-3 + 8*k;
yn1_1 = -0.8e-3 - 8*k;
yn2_1 = 0.8e-3 + 8*k;
a_xp_1 = 9*g;  
a_xn_1 = -9*g;

k_yp_1 = 1/(4*pi*((a_xp_1-x_new)^2+z_new^2));
k_1yp_1 = (yp2_1-y_new)/((yp2_1-y_new)^2+(a_xp_1-x_new)^2+z_new^2)^0.5;
k_2yp_1 = (yp1_1-y_new)/((yp1_1-y_new)^2+(a_xp_1-x_new)^2+z_new^2)^0.5;

k_1yp_3 = (yp2_1-y_new)/((yp2_1-y_new)^2+(a_xp_1-x_new)^2+z_new^2)^1.5;
k_2yp_3 = (yp1_1-y_new)/((yp1_1-y_new)^2+(a_xp_1-x_new)^2+z_new^2)^1.5;

k_yn_1 = 1/(4*pi*((a_xn_1-x_new)^2+z_new^2));
k_1yn_1 = (yn2_1-y_new)/((yn2_1-y_new)^2+(a_xn_1-x_new)^2+z_new^2)^0.5;
k_2yn_1 = (yn1_1-y_new)/((yn1_1-y_new)^2+(a_xn_1-x_new)^2+z_new^2)^0.5;

k_1yn_3 = (yn2_1-y_new)/((yn2_1-y_new)^2+(a_xn_1-x_new)^2+z_new^2)^1.5;
k_2yn_3 = (yn1_1-y_new)/((yn1_1-y_new)^2+(a_xn_1-x_new)^2+z_new^2)^1.5;


hyp_z_1 = (k_yp_1) *m0;
hyp_z1_1 = (k_1yp_1 - k_2yp_1)*(-1);
hyp_z2_1 = (k_yp_1*(k_1yp_1 - k_2yp_1)*(z_new^2))*4*pi*2;
hyp_z3_1 = (k_1yp_3 - k_2yp_3)*(z_new^2);
dxp_dz = hyp_z_1*(hyp_z1_1 + hyp_z2_1 + hyp_z3_1);


hyn_z_1 = (k_yn_1)* m0*(-1);
hyn_z1_1 = (k_1yn_1 - k_2yn_1)*(-1);
hyn_z2_1 = (k_yn_1*(k_1yn_1 - k_2yn_1)*(z_new^2))*4*pi*2;
hyn_z3_1 = (k_1yn_3 - k_2yn_3)*(z_new^2);
dxn_dz = hyn_z_1*(hyn_z1_1 + hyn_z2_1 + hyn_z3_1);

%--------%--------%--------%--------%--------%--------%--------%----------
% Line along x - axis
%-%--------%--------%--------%--------%a--------%--------%--------%--------
xp1_1 = -0.8e-3 - 8*k;
xp2_1 = 0.8e-3 + 8*k;
xn1_1 = -1e-3 - 8*k;
xn2_1 = 1e-3 + 8*k;
a_yp_1 = 3.875;          %Distance of coil from (0,0)
a_yn_1 = -3.875;

k_xp_1 = 1/(4*pi*((a_yp_1-y_new)^2+z_new^2));
k_1xp_1 = (xp2_1-x_new)/((xp2_1-x_new)^2+(a_yp_1-y_new)^2+z_new^2)^0.5;
k_2xp_1 = (xp1_1-x_new)/((xp1_1-x_new)^2+(a_yp_1-y_new)^2+z_new^2)^0.5;

k_xn_1 = 1/(4*pi*((a_yn_1-y_new)^2+z_new^2));
k_1xn_1 = (xn2_1-x_new)/((xn2_1-x_new)^2+(a_yn_1-y_new)^2+z_new^2)^0.5;
k_2xn_1 = (xn1_1-x_new)/((xn1_1-x_new)^2+(a_yn_1-y_new)^2+z_new^2)^0.5;

k_1xp_3 = (xp2_1-x_new)/((xp2_1-x_new)^2+(a_yp_1-y_new)^2+z_new^2)^1.5;
k_2xp_3 = (xp1_1-x_new)/((xp1_1-x_new)^2+(a_yp_1-y_new)^2+z_new^2)^1.5;

k_1xn_3 = (xn2_1-x_new)/((xn2_1-x_new)^2+(a_yn_1-y_new)^2+z_new^2)^1.5;
k_2xn_3 = (xn1_1-x_new)/((xn1_1-x_new)^2+(a_yn_1-y_new)^2+z_new^2)^1.5;


hxp_z_1 = (k_xp_1)*m0;
hxp_z1_1 = (k_1xp_1 - k_2xp_1)*(-1);
hxp_z2_1 = (k_xp_1*(k_1xp_1 - k_2xp_1)*(z_new^2))*4*pi*2;
hxp_z3_1 = (k_1xp_3 - k_2xp_3)*(z_new^2);
dyp_dz = hxp_z_1*(hxp_z1_1 + hxp_z2_1 + hxp_z3_1);


hxn_z_1 = (k_xn_1)*m0*(-1);
hxn_z1_1 = (k_1xn_1 - k_2xn_1)*(-1);
hxn_z2_1 = (k_xn_1*(k_1xn_1 - k_2xn_1)*(z_new^2))*4*pi*2;
hxn_z3_1 = (k_1xn_3 - k_2xn_3)*(z_new^2);
dyn_dz = hxn_z_1*(hxn_z1_1 + hxn_z2_1 + hxn_z3_1);

end

== matlab function I_for_8_coils_diagonal_motion/Right_Up_Coil/Left_Coil1/Inner 5 Coils/Coil-1 ==
  data: dxp_dz output; x_new input; y_new input; z_new input; dxn_dz output; dyp_dz output; dyn_dz output
function  [dxp_dz, dxn_dz, dyp_dz, dyn_dz] = current(x_new, y_new, z_new)

g = 520e-6;     %Coil spacing
m0 = 4*pi*1e-7;
radius = 3e-3;%m
height = 1e-3;%m
Magentization = 1.45; %T
vol_cy = pi*radius^2*height; % If Object is Cylinder, vol in m^3
% vol_sp = (4/3)*(pi * radius^3); % If Object is Sphere, vol in m^3

k = 0.4e-3; %additional length added to wires, to get concentric coil
%--------%--------%--------%--------%--------%--------%--------%----------
% Line along y - axis
%-%--------%--------%--------%--------%--------%--------%--------%--------
yp1_1 = -0.6e-3 ;
yp2_1 = 0.6e-3 ;
yn1_1 = -0.8e-3 ;
yn2_1 = 0.8e-3;
a_xp_1 = g;  
a_xn_1 = -g;

k_yp_1 = 1/(4*pi*((a_xp_1-x_new)^2+z_new^2));
k_1yp_1 = (yp2_1-y_new)/((yp2_1-y_new)^2+(a_xp_1-x_new)^2+z_new^2)^0.5;
k_2yp_1 = (yp1_1-y_new)/((yp1_1-y_new)^2+(a_xp_1-x_new)^2+z_new^2)^0.5;

k_1yp_3 = (yp2_1-y_new)/((yp2_1-y_new)^2+(a_xp_1-x_new)^2+z_new^2)^1.5;
k_2yp_3 = (yp1_1-y_new)/((yp1_1-y_new)^2+(a_xp_1-x_new)^2+z_new^2)^1.5;

k_yn_1 = 1/(4*pi*((a_xn_1-x_new)^2+z_new^2));
k_1yn_1 = (yn2_1-y_new)/((yn2_1-y_new)^2+(a_xn_1-x_new)^2+z_new^2)^0.5;
k_2yn_1 = (yn1_1-y_new)/((yn1_1-y_new)^2+(a_xn_1-x_new)^2+z_new^2)^0.5;

k_1yn_3 = (yn2_1-y_new)/((yn2_1-y_new)^2+(a_xn_1-x_new)^2+z_new^2)^1.5;
k_2yn_3 = (yn1_1-y_new)/((yn1_1-y_new)^2+(a_xn_1-x_new)^2+z_new^2)^1.5;


hyp_z_1 = (k_yp_1) *m0;
hyp_z1_1 = (k_1yp_1 - k_2yp_1)*(-1);
hyp_z2_1 = (k_yp_1*(k_1yp_1 - k_2yp_1)*(z_new^2))*4*pi*2;
hyp_z3_1 = (k_1yp_3 - k_2yp_3)*(z_new^2);
dxp_dz = hyp_z_1*(hyp_z1_1 + hyp_z2_1 + hyp_z3_1);


hyn_z_1 = (k_yn_1)* m0*(-1);
hyn_z1_1 = (k_1yn_1 - k_2yn_1)*(-1);
hyn_z2_1 = (k_yn_1*(k_1yn_1 - k_2yn_1)*(z_new^2))*4*pi*2;
hyn_z3_1 = (k_1yn_3 - k_2yn_3)*(z_new^2);
dxn_dz = hyn_z_1*(hyn_z1_1 + hyn_z2_1 + hyn_z3_1);

%--------%--------%--------%--------%--------%--------%--------%----------
% Line along x - axis
%-%--------%--------%--------%--------%a--------%--------%--------%--------
xp1_1 = -0.8e-3 ;
xp2_1 = 0.8e-3 ;
xn1_1 = -1e-3 ;
xn2_1 = 1e-3 ;
a_yp_1 = 0.675;          %Distance of coil from (0,0)
a_yn_1 = -0.675;

k_xp_1 = 1/(4*pi*((a_yp_1-y_new)^2+z_new^2));
k_1xp_1 = (xp2_1-x_new)/((xp2_1-x_new)^2+(a_yp_1-y_new)^2+z_new^2)^0.5;
k_2xp_1 = (xp1_1-x_new)/((xp1_1-x_new)^2+(a_yp_1-y_new)^2+z_new^2)^0.5;

k_xn_1 = 1/(4*pi*((a_yn_1-y_new)^2+z_new^2));
k_1xn_1 = (xn2_1-x_new)/((xn2_1-x_new)^2+(a_yn_1-y_new)^2+z_new^2)^0.5;
k_2xn_1 = (xn1_1-x_new)/((xn1_1-x_new)^2+(a_yn_1-y_new)^2+z_new^2)^0.5;

k_1xp_3 = (xp2_1-x_new)/((xp2_1-x_new)^2+(a_yp_1-y_new)^2+z_new^2)^1.5;
k_2xp_3 = (xp1_1-x_new)/((xp1_1-x_new)^2+(a_yp_1-y_new)^2+z_new^2)^1.5;

k_1xn_3 = (xn2_1-x_new)/((xn2_1-x_new)^2+(a_yn_1-y_new)^2+z_new^2)^1.5;
k_2xn_3 = (xn1_1-x_new)/((xn1_1-x_new)^2+(a_yn_1-y_new)^2+z_new^2)^1.5;


hxp_z_1 = (k_xp_1)*m0;
hxp_z1_1 = (k_1xp_1 - k_2xp_1)*(-1);
hxp_z2_1 = (k_xp_1*(k_1xp_1 - k_2xp_1)*(z_new^2))*4*pi*2;
hxp_z3_1 = (k_1xp_3 - k_2xp_3)*(z_new^2);
dyp_dz = hxp_z_1*(hxp_z1_1 + hxp_z2_1 + hxp_z3_1);


hxn_z_1 = (k_xn_1)*m0*(-1);
hxn_z1_1 = (k_1xn_1 - k_2xn_1)*(-1);
hxn_z2_1 = (k_xn_1*(k_1xn_1 - k_2xn_1)*(z_new^2))*4*pi*2;
hxn_z3_1 = (k_1xn_3 - k_2xn_3)*(z_new^2);
dyn_dz = hxn_z_1*(hxn_z1_1 + hxn_z2_1 + hxn_z3_1);

end
